simulink model "DYN_02x"  (R2021a)
settings: Solver=FixedStepAuto  StartTime=0.0  StopTime=50  FixedStep=0.001  RelTol=1e-3
(part 1 of 53)
settings Model: Creator=TMP  LastModifiedBy=TMP
settings SolverCC: AlgebraicLoopSolver=TrustRegion
settings DebuggingCC: SFMachineParentedDataDiag=warning

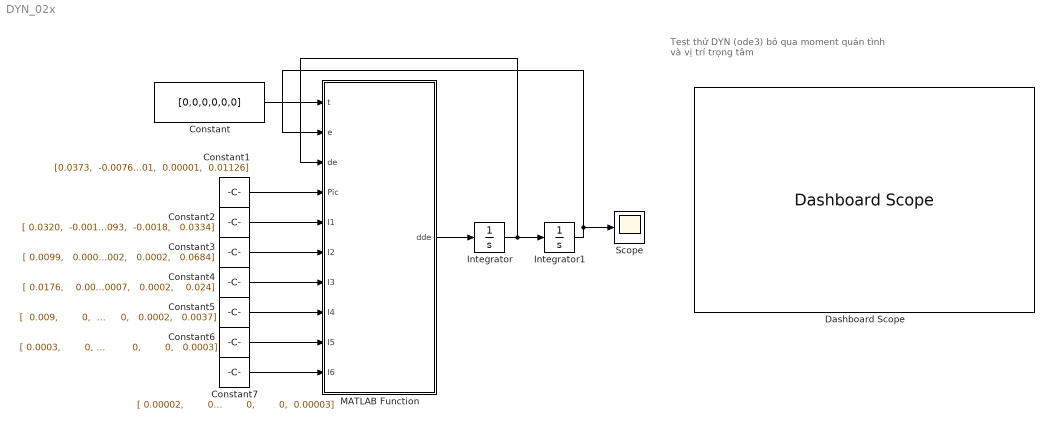
== system DYN_02x ==
  note: Test thử DYN (ode3)
      | bỏ qua moment quán tình và vị trí trọng tâm
  Constant : Constant  Value=[0,0,0,0,0,0]
  Constant1 : Constant  Value=|
      | [0.0373,  -0.0076,   0.1064;
      |        0.1127,   0.0065,   0.0648;
      |        0.0447,   0.0125,  -0.0554;
      |        0.0006,   0.0052,   0.1068;
      |             0,   0.0062,   0.0195;
      |      -0.00001,  0.00001,  0.01126]
  Constant2 : Constant  Value=|
      | [ 0.0320,  -0.0017,   0.0093;
      |       -0.0017,   0.0364,  -0.0018;
      |        0.0093,  -0.0018,   0.0334]
  Constant3 : Constant  Value=|
      | [ 0.0099,   0.0008,  -0.0002;
      |        0.0008,   0.0646,   0.0002;
      |       -0.0002,   0.0002,   0.0684]
  Constant4 : Constant  Value=|
      | [ 0.0176,    0.001,   0.0007;
      |         0.001,   0.0195,   0.0002;
      |        0.0007,   0.0002,    0.024]
  Constant5 : Constant  Value=|
      | [  0.009,        0,        0;
      |             0,   0.0081,   0.0002;
      |             0,   0.0002,   0.0037]
  Constant6 : Constant  Value=|
      | [ 0.0003,        0,        0;
      |             0,   0.0002,        0;
      |             0,        0,   0.0003]
  Constant7 : Constant  Value=|
      | [ 0.00002,        0,        0;
      |              0,  0.00002,        0;
      |              0,        0,  0.00003]
  Dashboard Scope : DashboardScope
  Integrator : Integrator  InitialCondition=[0.2;0.2;0.2;0.2;0.2;0.2]
  Integrator1 : Integrator  InitialCondition=[0.1;0.1;0.1;0.1;0.1;0.1]
  MATLAB Function : MATLAB Function  TreatAsAtomicUnit=on
  Scope : Scope
  wires:
  MATLAB Function/1(dde) -> Integrator/1
  Integrator/1 -> MATLAB Function/3(de), Integrator1/1
  Integrator1/1 -> MATLAB Function/2(e), Scope/1
  Constant/1 -> MATLAB Function/1(t)
  Constant1/1 -> MATLAB Function/4(Pic)
  Constant2/1 -> MATLAB Function/5(I1)
  Constant3/1 -> MATLAB Function/6(I2)
  Constant4/1 -> MATLAB Function/7(I3)
  Constant5/1 -> MATLAB Function/8(I4)
  Constant6/1 -> MATLAB Function/9(I5)
  Constant7/1 -> MATLAB Function/10(I6)
